simulink library "Lib_PFSys_BiDirBattery_TMATS"  (R2017a)
settings: Solver=ode45  StartTime=0.0  StopTime=10.0  RelTol=1e-3  EnableMultiTasking=on
libraries: Lib_PF_LineDC_TMATS x1, Lib_PF_BusLoadDC_TMATS x1, Lib_PF_BusSlackDC_TMATS x1
Description:
  | Thomas Modules
settings Model: Creator=jwchapm2  LastModifiedBy=glthoma1
settings DataIOCC: LimitDataPoints=on  SaveFormat=Array
settings OptimizationCC: ExpressionDepthLimit=2147483647  LifeSpan=inf
settings DebuggingCC: UnderspecifiedInitializationDetection=Classic  MergeDetectMultiDrivingBlocksExec=none  SolverPrmCheckMsg=warning  StateNameClashWarn=warning  SFUnexpectedBacktrackingDiag=warning  SFNoUnconditionalDefaultTransitionDiag=warning  SFExecutionAtInitializationDiag=none
settings HardwareCC: ProdBitPerPointer=32  ProdBitPerSizeT=32  ProdBitPerPtrDiffT=32  ProdLargestAtomicFloat=None  ProdIntDivRoundTo=Undefined  ProdEndianess=Unspecified  ProdWordSize=32  ProdHWDeviceType=32-bit Generic
settings ModelReferenceCC: PropagateSignalLabelsOutOfModel=off
settings GRTTargetCC: TargetLangStandard=C89/C90 (ANSI)  GeneratePreprocessorConditionals=Disable all
settings ConfigComp: CovMetricSettings=dw  CovHtmlReporting=on  CovSaveCumulativeToWorkspaceVar=on  CovSaveSingleToWorkspaceVar=on  CovExternalEMLEnable=off

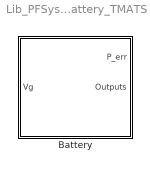
== system Lib_PFSys_BiDirBattery_TMATS ==
  "Battery " : Subsystem  mask(Battery){V_M=475, Z_M=0.001}
      mask prompts: V_M "V_M - Nominal Voltage"; Z_M "Z_M - Impedance"
      mask help: This block represents a battery with a specified nominal voltage and internal impedance.

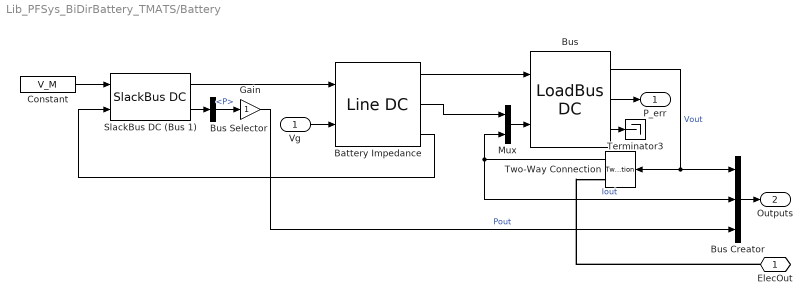
== system Lib_PFSys_BiDirBattery_TMATS/Battery  ==
  Vg : Inport
  Battery Impedance : Lib_PF_LineDC_TMATS/Line DC  R_M=Z_M
  Bus : Lib_PF_BusLoadDC_TMATS/LoadBus DC  PeInEN_M=off  P_M=0  BlkNm_M=double(gcb)
  Bus Creator : BusCreator  Inputs=3
  Bus Selector : BusSelector  OutputSignals=P
  Constant : Constant  Value=V_M
  Gain : Gain
  Mux : Mux  Inputs=2
  SlackBus DC (Bus 1) : Lib_PF_BusSlackDC_TMATS/SlackBus DC
  Terminator3 : Terminator
  Two-Way Connection : TwoWayConnection
  ElecOut : PMIOPort  Port=1  Side=Right
  P_err : Outport
  Outputs : Outport  Port=2
  wires:
  Battery Impedance/2 -> Mux/1
  Gain/1 -> Bus Creator/3  "Pout"
  Bus Selector/1 -> Gain/1  "<P>"
  Bus Creator/1 -> Outputs/1
  Two-Way Connection/1 -> Mux/2, Bus Creator/2  "Iout"
  Mux/1 -> Bus/2
  Battery Impedance/3 -> SlackBus DC (Bus 1)/2
  Bus/2 -> P_err/1
  Constant/1 -> SlackBus DC (Bus 1)/1
  SlackBus DC (Bus 1)/2 -> Bus Selector/1
  Bus/3 -> Terminator3/1
  Bus/1 -> Two-Way Connection/1, Bus Creator/1  "Vout"
  Battery Impedance/1 -> Bus/1
  SlackBus DC (Bus 1)/1 -> Battery Impedance/1
  Vg/1 -> Battery Impedance/2
  connections:
  ElecOut/RConn1 -- Two-Way Connection/RConn1
